simulink model "Quadcopter"  (R2019a)
settings: Solver=VariableStepAuto  StartTime=0.0  StopTime=2000  MaxStep=1e-1  RelTol=1e-3
StopFcn:
  | hold on;
  | plot3(out.out_y1.data, out.out_x1.data, out.out_z1.data, 'r');
  | plot3(out.out_y2.data, out.out_x2.data, out.out_z2.data, 'g');
  | plot3(out.out_y3.data, out.out_x3.data, out.out_z3.data, 'b');
  | plot3([0;out.out_y.data(1:1000:end)], [0;out.out_x.data(1:1000:end)], [0;out.out_z.data(1:1000:end)], '.k');
  | view(3);
  | hold off;
values from neighbouring files (symbols this model uses):
  B_phi = 1    [Control.m]
  B_psi = 1    [Control.m]
  B_theta = 1    [Control.m]
  B_z = 5    [Control.m]
  r_x12 = 8    [Control.m]
  r_x32 = 4    [Control.m]
  r_y12 = 8    [Control.m]
  r_y32 = 4    [Control.m]
undefined symbols (not defined in the file or in its folder): As, Bs, Cpsi, Cs, Cx, Cy, Cz, Ds, x01, x02, x03, y01, y02, y03, z01, z02, z03
libraries: simulink x1
(part 1 of 3)
settings Model: Creator=hvh  LastModifiedBy=hvh

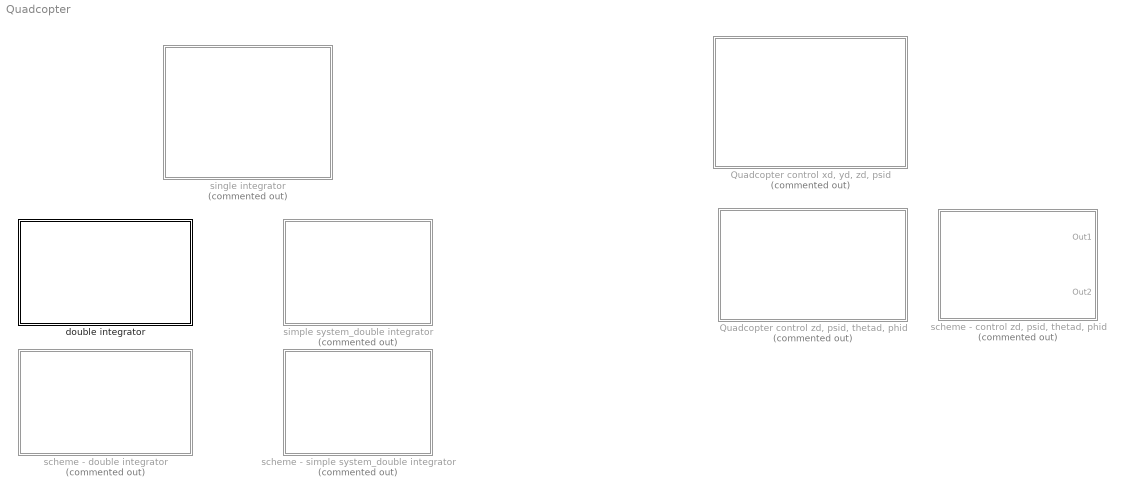
== system Quadcopter ==
  "Quadcopter control xd, yd, zd, psid" : Subsystem  Commented=on
  "Quadcopter control zd, psid, thetad, phid" : Subsystem  Commented=on
  double integrator : Subsystem
  "scheme - control zd, psid, thetad, phid" : Subsystem  Commented=on
  scheme - double integrator : Subsystem  Commented=on
  scheme - simple system_double integrator : Subsystem  Commented=on
  simple system_double integrator : Subsystem  Commented=on
  single integrator : Subsystem  Commented=on

== system Quadcopter/Quadcopter control xd, yd, zd, psid ==
  Controller : Subsystem
  Demux : Demux  Outputs=6
  Demux1 : Demux  Outputs=6
  Dynamic_System : Subsystem
  Mux : Mux  Inputs=6
  Mux1 : Mux  Inputs=6
  psi - psid : Scope  NumInputPorts=2
  psid : Step  Time=0  After=0.1  SampleTime=0
  x - xd : Scope  NumInputPorts=2
  xd : Step  Time=0  After=3  SampleTime=0
  y - yd : Scope  NumInputPorts=2
  yd : Step  Time=0  After=6  SampleTime=0
  z - zd : Scope  NumInputPorts=2
  zd : Step  Time=0  After=20  SampleTime=0
  wires:
  Dynamic_System/11(psi) -> Mux1/5
  Controller/4(tau_psi) -> Dynamic_System/4(tau_psi)
  Dynamic_System/3(y) -> Mux/3
  Dynamic_System/1(x) -> Mux/1
  Controller/2(tau_phi) -> Dynamic_System/2(tau_phi)
  Dynamic_System/5(z) -> Mux/5
  Controller/3(tau_theta) -> Dynamic_System/3(tau_theta)
  Controller/1(Ft) -> Dynamic_System/1(Ft)
  Dynamic_System/2(dx) -> Mux/2
  Dynamic_System/4(dy) -> Mux/4
  Dynamic_System/6(dz) -> Mux/6
  Dynamic_System/7(phi) -> Mux1/1
  Dynamic_System/8(dphi) -> Mux1/2
  Dynamic_System/9(theta) -> Mux1/3
  Dynamic_System/10(dtheta) -> Mux1/4
  Dynamic_System/12(dpsi) -> Mux1/6
  Demux/1 -> x - xd/1, Controller/1(x)
  Demux/2 -> Controller/2(dx)
  Demux/3 -> y - yd/1, Controller/3(y)
  Demux/4 -> Controller/4(dy)
  Demux/5 -> Controller/5(z), z - zd/1
  Demux/6 -> Controller/6(dz)
  Mux/1 -> Demux/1
  Demux1/2 -> Controller/8(dphi)
  Demux1/3 -> Controller/9(theta)
  Demux1/4 -> Controller/10(dtheta)
  Demux1/5 -> psi - psid/1, Controller/11(psi)
  Demux1/6 -> Controller/12(dpsi)
  Mux1/1 -> Demux1/1
  xd/1 -> x - xd/2, Controller/13(xd)
  yd/1 -> y - yd/2, Controller/14(yd)
  zd/1 -> z - zd/2, Controller/15(zd)
  psid/1 -> psi - psid/2, Controller/16(psid)
  Demux1/1 -> Controller/7(phi)

== system Quadcopter/Quadcopter control zd, psid, thetad, phid ==
  Controller : Subsystem
  Demux : Demux  Outputs=8
  Dynamic_System : Subsystem
  Mux : Mux  Inputs=8
  ddx : Scope
  ddy : Scope
  dphid : Step  Time=0  After=0  SampleTime=0
  dthetad : Step  Time=0  After=0  SampleTime=0
  dx : Scope
  dy : Scope
  phi : Scope  NumInputPorts=2
  phid : Step  Time=0  After=0.1  SampleTime=0
  psi : Scope  NumInputPorts=2
  psid : Step  Time=0  After=0.1  SampleTime=0
  theta : Scope  NumInputPorts=2
  thetad : Step  Time=0  After=0.15  SampleTime=0
  x : Scope
  y : Scope
  z : Scope  NumInputPorts=2
  zd : Step  Time=0  SampleTime=0
  wires:
  Dynamic_System/3(psi) -> Mux/3, psi/2
  Controller/4(tau_psi) -> Dynamic_System/4(tau_psi)
  Dynamic_System/12(y) -> y/1
  Dynamic_System/9(x) -> x/1
  Controller/2(tau_phi) -> Dynamic_System/2(tau_phi)
  Controller/3(tau_theta) -> Dynamic_System/3(tau_theta)
  Controller/1(Ft) -> Dynamic_System/1(Ft)
  Dynamic_System/10(dx) -> dx/1
  Dynamic_System/13(dy) -> dy/1
  Mux/1 -> Demux/1
  zd/1 -> z/1, Controller/9(zd)
  psid/1 -> psi/1, Controller/10(psid)
  phid/1 -> Controller/13(phid), phi/1
  dphid/1 -> Controller/14(dphid)
  thetad/1 -> Controller/11(thetad), theta/1
  dthetad/1 -> Controller/12(dthetad)
  Dynamic_System/11(ddx) -> ddx/1
  Dynamic_System/14(ddy) -> ddy/1
  Dynamic_System/1(z) -> z/2, Mux/1
  Dynamic_System/2(dz) -> Mux/2
  Dynamic_System/4(dpsi) -> Mux/4
  Dynamic_System/5(theta) -> theta/2, Mux/5
  Dynamic_System/6(dtheta) -> Mux/6
  Dynamic_System/8(dphi) -> Mux/8
  Dynamic_System/7(phi) -> Mux/7, phi/2
  Demux/1 -> Controller/1(z)
  Demux/2 -> Controller/2(dz)
  Demux/3 -> Controller/3(psi)
  Demux/4 -> Controller/4(dpsi)
  Demux/5 -> Controller/5(theta)
  Demux/6 -> Controller/6(dtheta)
  Demux/7 -> Controller/7(phi)
  Demux/8 -> Controller/8(dphi)

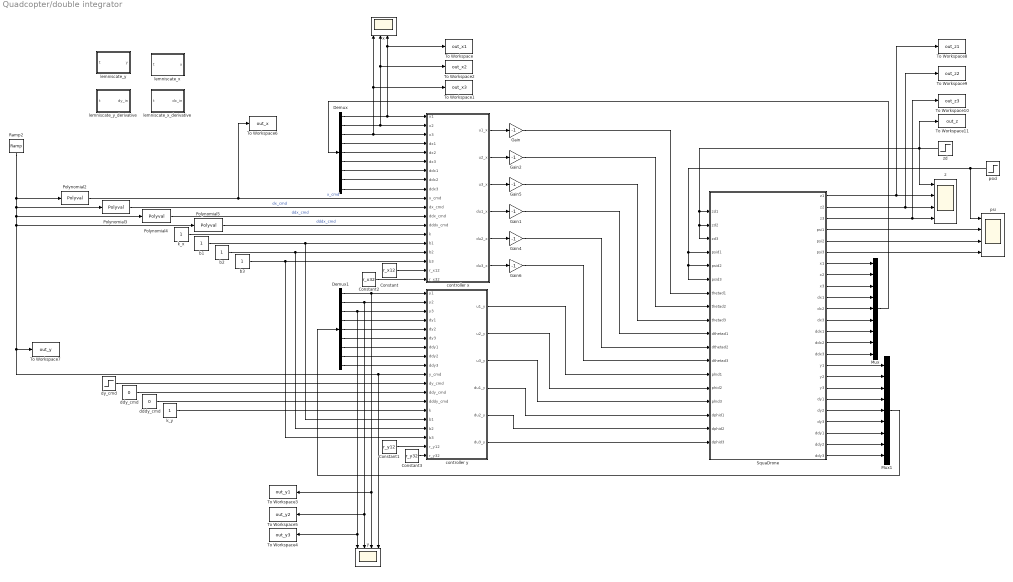
== system Quadcopter/double integrator ==
  Constant : Constant  Value=r_x12
  Constant1 : Constant  Value=r_y12
  Constant2 : Constant  Value=r_x32
  Constant3 : Constant  Value=r_y32
  Demux : Demux  Outputs=9
  Demux1 : Demux  Outputs=9
  Gain{,1..2,4..6} (6 alike) : Gain  Gain=-1
  Mux : Mux  Inputs=9
  Mux1 : Mux  Inputs=9
  Polynomial2 : Polyval  Coefs=[2*1e-5 -0.5*1e-2 0 0]
  Polynomial3 : Polyval  Coefs=[6*1e-5 -1e-2 0]
  Polynomial4 : Polyval  Coefs=[12*1e-5 -1e-2]
  Polynomial5 : Polyval  Coefs=[12*1e-5]
  Ramp2 : simulink/Sources/Ramp  slope=1/10  start=15  InitialOutput=0
  SquaDrone : Subsystem
  To Workspace : ToWorkspace  VariableName=out_x1  SaveFormat=Timeseries  SampleTime=-1
  To Workspace1 : ToWorkspace  VariableName=out_x3  SaveFormat=Timeseries  SampleTime=-1
  To Workspace10 : ToWorkspace  VariableName=out_z3  SaveFormat=Timeseries  SampleTime=-1
  To Workspace11 : ToWorkspace  VariableName=out_z  SaveFormat=Timeseries  SampleTime=-1
  To Workspace2 : ToWorkspace  VariableName=out_x2  SaveFormat=Timeseries  SampleTime=-1
  To Workspace3 : ToWorkspace  VariableName=out_y1  SaveFormat=Timeseries  SampleTime=-1
  To Workspace4 : ToWorkspace  VariableName=out_y3  SaveFormat=Timeseries  SampleTime=-1
  To Workspace5 : ToWorkspace  VariableName=out_y2  SaveFormat=Timeseries  SampleTime=-1
  To Workspace6 : ToWorkspace  VariableName=out_x  SaveFormat=Timeseries  SampleTime=-1
  To Workspace7 : ToWorkspace  VariableName=out_y  SaveFormat=Timeseries  SampleTime=-1
  To Workspace8 : ToWorkspace  VariableName=out_z1  SaveFormat=Timeseries  SampleTime=-1
  To Workspace9 : ToWorkspace  VariableName=out_z2  SaveFormat=Timeseries  SampleTime=-1
  b1 : Constant
  b2 : Constant
  b3 : Constant
  controller x : MATLAB Function  TreatAsAtomicUnit=on
  controller y : MATLAB Function  TreatAsAtomicUnit=on
  dddy_cmd : Constant  Value=0
  ddy_cmd : Constant  Value=0
  dy_cmd : Step  Time=15  SampleTime=0
  k_x : Constant
  k_y : Constant
  lemniscate_x : MATLAB Function  TreatAsAtomicUnit=on
  lemniscate_x_derivative : MATLAB Function  TreatAsAtomicUnit=on
  "lemniscate_y " : MATLAB Function  TreatAsAtomicUnit=on
  "lemniscate_y_derivative " : MATLAB Function  TreatAsAtomicUnit=on
  psi : Scope  NumInputPorts=4
  psid : Step  Time=0  After=0  SampleTime=0
  x : Scope  NumInputPorts=4
  y : Scope  NumInputPorts=4
  z : Scope  NumInputPorts=4
  zd : Step  Time=0  After=10  SampleTime=0
  wires:
  b2/1 -> controller x/16(b2), controller y/16(b2)
  b3/1 -> controller y/17(b3), controller x/17(b3)
  b1/1 -> controller x/15(b1), controller y/15(b1)
  k_x/1 -> controller x/14(k)
  controller x/1(u1_x) -> Gain/1
  controller x/4(du1_x) -> Gain1/1
  controller x/2(u2_x) -> Gain2/1
  controller x/5(du2_x) -> Gain4/1
  controller x/3(u3_x) -> Gain5/1
  controller x/6(du3_x) -> Gain6/1
  zd/1 -> To Workspace11/1, z/1, SquaDrone/3(zd3), SquaDrone/2(zd2), SquaDrone/1(zd1)
  psid/1 -> SquaDrone/6(psid3), SquaDrone/5(psid2), SquaDrone/4(psid1), psi/1
  Demux/5 -> controller x/5(dx2)
  Demux/6 -> controller x/6(dx3)
  Demux/8 -> controller x/8(ddx2)
  Demux/7 -> controller x/7(ddx1)
  Demux/9 -> controller x/9(ddx3)
  Demux1/4 -> controller y/4(dy1)
  Demux1/5 -> controller y/5(dy2)
  Demux1/6 -> controller y/6(dy3)
  Demux1/7 -> controller y/7(ddy1)
  Demux1/8 -> controller y/8(ddy2)
  Demux1/9 -> controller y/9(ddy3)
  Mux/1 -> Demux/1
  Demux/4 -> controller x/4(dx1)
  SquaDrone/10(dx1) -> Mux/4
  SquaDrone/11(dx2) -> Mux/5
  SquaDrone/12(dx3) -> Mux/6
  SquaDrone/13(ddx1) -> Mux/7
  SquaDrone/14(ddx2) -> Mux/8
  SquaDrone/15(ddx3) -> Mux/9
  SquaDrone/7(x1) -> Mux/1
  SquaDrone/8(x2) -> Mux/2
  SquaDrone/9(x3) -> Mux/3
  SquaDrone/23(ddy2) -> Mux1/8
  SquaDrone/24(ddy3) -> Mux1/9
  SquaDrone/22(ddy1) -> Mux1/7
  SquaDrone/21(dy3) -> Mux1/6
  SquaDrone/20(dy2) -> Mux1/5
  SquaDrone/19(dy1) -> Mux1/4
  SquaDrone/16(y1) -> Mux1/1
  SquaDrone/17(y2) -> Mux1/2
  SquaDrone/18(y3) -> Mux1/3
  Mux1/1 -> Demux1/1
  Demux/2 -> controller x/2(x2), x/2, To Workspace2/1
  Demux/3 -> controller x/3(x3), x/1, To Workspace1/1
  Demux/1 -> controller x/1(x1), x/3, To Workspace/1
  SquaDrone/6(psi3) -> psi/4
  SquaDrone/5(psi2) -> psi/3
  SquaDrone/4(psi1) -> psi/2
  SquaDrone/1(z1) -> To Workspace8/1, z/2
  SquaDrone/2(z2) -> To Workspace9/1, z/3
  SquaDrone/3(z3) -> To Workspace10/1, z/4
  Demux1/1 -> y/3, To Workspace3/1, controller y/1(y1)
  Demux1/2 -> y/2, To Workspace5/1, controller y/2(y2)
  Demux1/3 -> To Workspace4/1, y/1, controller y/3(y3)
  controller y/6(du3_y) -> SquaDrone/18(dphid3)
  controller y/5(du2_y) -> SquaDrone/17(dphid2)
  controller y/4(du1_y) -> SquaDrone/16(dphid1)
  controller y/3(u3_y) -> SquaDrone/15(phid3)
  controller y/2(u2_y) -> SquaDrone/14(phid2)
  controller y/1(u1_y) -> SquaDrone/13(phid1)
  Gain6/1 -> SquaDrone/12(dthetad3)
  Gain4/1 -> SquaDrone/11(dthetad2)
  Gain1/1 -> SquaDrone/10(dthetad1)
  Gain5/1 -> SquaDrone/9(thetad3)
  Gain2/1 -> SquaDrone/8(thetad2)
  Gain/1 -> SquaDrone/7(thetad1)
  Constant/1 -> controller x/18(r_x12)
  Constant1/1 -> controller y/18(r_y12)
  Constant2/1 -> controller x/19(r_x32)
  Constant3/1 -> controller y/19(r_y32)
  k_y/1 -> controller y/14(k)
  dy_cmd/1 -> controller y/11(dy_cmd)
  ddy_cmd/1 -> controller y/12(ddy_cmd)
  Polynomial2/1 -> To Workspace6/1, controller x/10(x_cmd)  "x_cmd"
  Polynomial3/1 -> controller x/11(dx_cmd)  "dx_cmd"
  Polynomial5/1 -> controller x/13(dddx_cmd)  "dddx_cmd"
  Polynomial4/1 -> controller x/12(ddx_cmd)  "ddx_cmd"
  Ramp2/1 -> To Workspace7/1, controller y/10(y_cmd), y/4, Polynomial5/1, Polynomial4/1, Polynomial3/1, Polynomial2/1
  dddy_cmd/1 -> controller y/13(dddy_cmd)

== system Quadcopter/scheme - control zd, psid, thetad, phid ==
  Controller : Subsystem
  Demux2 : Demux
  Desired input : Subsystem
  Drone : Subsystem
  Mux2 : Mux
  Out1 : Outport
  Out2 : Outport  Port=2
  wires:
  Demux2/1 -> Controller/1(In1)  "Z"
  Controller/1(Out1) -> Drone/1(In1)  "Ft"
  Controller/2(Out2) -> Drone/2(In2)  "tau_psi"
  Drone/4(Output3) -> Mux2/4  "PHI"
  Demux2/2 -> Controller/2(In2)  "PSI"
  Drone/1(Output) -> Mux2/1  "Z"
  Mux2/1 -> Demux2/1
  Demux2/3 -> Controller/3(In3)  "THETA"
  Controller/3(Out3) -> Drone/3(In3)  "tau_theta"
  Drone/3(Output2) -> Mux2/3  "THETA"
  Demux2/4 -> Controller/4(In4)  "PHI"
  Drone/2(Output1) -> Mux2/2  "PSI"
  Controller/4(Out4) -> Drone/4(In4)  "thau_phi"
  Drone/5(Output4) -> Out1/1  "X"
  Drone/6(Output5) -> Out2/1  "Y"
  Desired input/1(Out1) -> Controller/5(In5)  "Z_d"
  Desired input/2(Out2) -> Controller/6(In6)  "PSI_d"
  Desired input/3(Out3) -> Controller/7(In7)  "THETA_d"
  Desired input/4(Out4) -> Controller/8(In8)  "PHI_d"

== system Quadcopter/scheme - double integrator ==
  "Change input from (X,Y) to (THETA, PHI)" : MATLAB Function  TreatAsAtomicUnit=on
  Coefficients : Subsystem
  Desired Inputs of X_d and Y_d : Subsystem
  Desired Inputs of Z_d and PSI_d : Subsystem
  Distances : Subsystem
  SquaDrone : Subsystem
  controller x : MATLAB Function  TreatAsAtomicUnit=on
  controller y : MATLAB Function  TreatAsAtomicUnit=on
  wires:
  Desired Inputs of X_d and Y_d/1(X_d) -> controller x/2(X_dX_ddX_ddX_cmd)
  Desired Inputs of X_d and Y_d/2(Y_d) -> controller y/2(Y_dY_ddY_ddY_cmd)
  Coefficients/2(Coef_Y) -> controller y/3(k_b1_b2_b3)
  Coefficients/1(Coef_X) -> controller x/3(k_b1_b2_b3)
  Distances/1(Distance_X) -> controller x/4(r)
  Distances/2(Distance_Y) -> controller y/4(r)
  "Change input from (X,Y) to (THETA, PHI)"/1(THETA_d) -> SquaDrone/3(THETA_d)
  "Change input from (X,Y) to (THETA, PHI)"/2(dTHETA_d) -> SquaDrone/4(dTHETA_d)
  "Change input from (X,Y) to (THETA, PHI)"/3(PHI_d) -> SquaDrone/5(PHI_d)
  "Change input from (X,Y) to (THETA, PHI)"/4(dPHI_d) -> SquaDrone/6(dPHI_d)
  controller x/1(U_x) -> "Change input from (X,Y) to (THETA, PHI)"/1(U_x)
  controller x/2(dU_x) -> "Change input from (X,Y) to (THETA, PHI)"/2(dU_x)
  controller y/1(U_Y) -> "Change input from (X,Y) to (THETA, PHI)"/3(U_y)
  controller y/2(dU_Y) -> "Change input from (X,Y) to (THETA, PHI)"/4(dU_y)
  Desired Inputs of Z_d and PSI_d/1(Z_d) -> SquaDrone/1(Z_d)
  Desired Inputs of Z_d and PSI_d/2(PSI_d) -> SquaDrone/2(PSI_d)
  SquaDrone/1(X_dX_ddX) -> controller x/1(X_dX_ddX)
  SquaDrone/2(Y_dY_ddY) -> controller y/1(Y_dY_ddY)

== system Quadcopter/scheme - simple system_double integrator ==
  Coefficients : Subsystem
  Demux : Demux  Outputs=6
  Desired Inputs : Subsystem
  Distances : Subsystem
  Mux : Mux  Inputs=6
  "Path Tracking Controller " : MATLAB Function  TreatAsAtomicUnit=on
  System Dynamics : Subsystem
  wires:
  "Path Tracking Controller "/2(u2) -> System Dynamics/2(u2)  "u2"
  "Path Tracking Controller "/1(u1) -> System Dynamics/1(u1)  "u1"
  "Path Tracking Controller "/3(u3) -> System Dynamics/3(u3)  "u3"
  Demux/1 -> "Path Tracking Controller "/1(x1)
  Demux/2 -> "Path Tracking Controller "/2(dx1)
  Demux/3 -> "Path Tracking Controller "/3(x2)
  Demux/4 -> "Path Tracking Controller "/4(dx2)
  Demux/5 -> "Path Tracking Controller "/5(x3)
  Demux/6 -> "Path Tracking Controller "/6(dx3)
  System Dynamics/1(x1) -> Mux/1
  System Dynamics/2(dx1) -> Mux/2
  System Dynamics/3(x2) -> Mux/3
  System Dynamics/4(dx2) -> Mux/4
  System Dynamics/5(x3) -> Mux/5
  System Dynamics/6(dx3) -> Mux/6
  Mux/1 -> Demux/1
  Desired Inputs/1(x_cmd) -> "Path Tracking Controller "/7(x_cmd)
  Desired Inputs/2(dx_cmd) -> "Path Tracking Controller "/8(dx_cmd)
  Coefficients/1(k) -> "Path Tracking Controller "/9(k)
  Coefficients/2(b1) -> "Path Tracking Controller "/10(b1)
  Coefficients/3(b2) -> "Path Tracking Controller "/11(b2)
  Coefficients/4(b3) -> "Path Tracking Controller "/12(b3)
  Distances/1(r_12) -> "Path Tracking Controller "/13(r_12)
  Distances/2(r_32) -> "Path Tracking Controller "/14(r_32)

== system Quadcopter/simple system_double integrator ==
  Demux : Demux  Outputs=6
  Dynamics : Subsystem
  MATLAB Function : MATLAB Function  TreatAsAtomicUnit=on
  Mux : Mux  Inputs=6
  b{1..3,5} (4 alike) : Constant
  b4 : Constant  Value=2
  dx_cmd : Step  Time=0  After=0  SampleTime=0
  k : Constant
  x : Scope  NumInputPorts=4
  x_cmd : Step  Time=0  After=0  SampleTime=0
  wires:
  MATLAB Function/2(u2) -> Dynamics/2(u2)
  MATLAB Function/1(u1) -> Dynamics/1(u1)
  MATLAB Function/3(u3) -> Dynamics/3(u3)
  x_cmd/1 -> x/1, MATLAB Function/7(x_cmd)
  dx_cmd/1 -> MATLAB Function/8(dx_cmd)
  k/1 -> MATLAB Function/9(k)
  b1/1 -> MATLAB Function/10(b1)
  b2/1 -> MATLAB Function/11(b2)
  b3/1 -> MATLAB Function/12(b3)
  b4/1 -> MATLAB Function/13(r_12)
  b5/1 -> MATLAB Function/14(r_32)
  Dynamics/1(x1) -> x/2, Mux/1
  Dynamics/2(dx1) -> Mux/2
  Dynamics/3(x2) -> x/3, Mux/3
  Dynamics/4(dx2) -> Mux/4
  Dynamics/5(x3) -> x/4, Mux/5
  Dynamics/6(dx3) -> Mux/6
  Demux/1 -> MATLAB Function/1(x1)
  Demux/2 -> MATLAB Function/2(dx1)
  Demux/3 -> MATLAB Function/3(x2)
  Demux/4 -> MATLAB Function/4(dx2)
  Demux/5 -> MATLAB Function/5(x3)
  Demux/6 -> MATLAB Function/6(dx3)
  Mux/1 -> Demux/1

== system Quadcopter/single integrator ==
  Constant : Constant
  Constant1 : Constant
  Demux : Demux  Outputs=3
  Demux1 : Demux  Outputs=3
  Formation dynamics x : StateSpace  A=As  B=Bs  C=Cs  D=Ds  InitialCondition=0
  Formation dynamics y : StateSpace  A=As  B=Bs  C=Cs  D=Ds  InitialCondition=0
  SquaDrone : Subsystem
  psi : Scope  NumInputPorts=3
  psid : Step  Time=0  After=0.1  SampleTime=0
  u1_x = f() : MATLAB Function  TreatAsAtomicUnit=on
  u1_y = f() : MATLAB Function  TreatAsAtomicUnit=on
  x : Scope  NumInputPorts=3
  x_cmd : Step  Time=0  After=10  SampleTime=0
  y : Scope  NumInputPorts=3
  y_cmd : Step  Time=0  After=15  SampleTime=0
  z : Scope  NumInputPorts=3
  zd : Step  Time=0  After=50  SampleTime=0
  wires:
  SquaDrone/8(psi2) -> psi/2
  SquaDrone/11(z3) -> z/3
  Demux/2 -> SquaDrone/5(x2d)
  psid/1 -> SquaDrone/12(psi3d), SquaDrone/8(psi2d), SquaDrone/4(psi1d)
  Demux1/3 -> SquaDrone/10(y3d)
  Demux/3 -> SquaDrone/9(x3d)
  SquaDrone/5(x2) -> x/2, u1_x = f()/2(x2)
  zd/1 -> SquaDrone/3(z1d), SquaDrone/7(z2d), SquaDrone/11(z3d)
  Demux1/1 -> SquaDrone/2(y1d)
  Constant/1 -> u1_y = f()/5(k), u1_x = f()/5(k)
  Constant1/1 -> u1_y = f()/6(b), u1_x = f()/6(b)
  SquaDrone/1(x1) -> x/3, u1_x = f()/1(x1)
  Formation dynamics x/1 -> Demux/1
  SquaDrone/9(x3) -> u1_x = f()/3(x3), x/1
  SquaDrone/2(y1) -> y/3, u1_y = f()/1(y1)
  x_cmd/1 -> u1_x = f()/4(x_cmd)
  SquaDrone/6(y2) -> y/2, u1_y = f()/2(y2)
  SquaDrone/10(y3) -> y/1, u1_y = f()/3(y3)
  y_cmd/1 -> u1_y = f()/4(y_cmd)
  SquaDrone/3(z1) -> z/1
  SquaDrone/7(z2) -> z/2
  Demux1/2 -> SquaDrone/6(y2d)
  u1_x = f()/1(u1_x) -> Formation dynamics x/1
  Formation dynamics y/1 -> Demux1/1
  Demux/1 -> SquaDrone/1(x1d)
  u1_y = f()/1(u1_y) -> Formation dynamics y/1
  SquaDrone/4(psi1) -> psi/1
  SquaDrone/12(psi3) -> psi/3

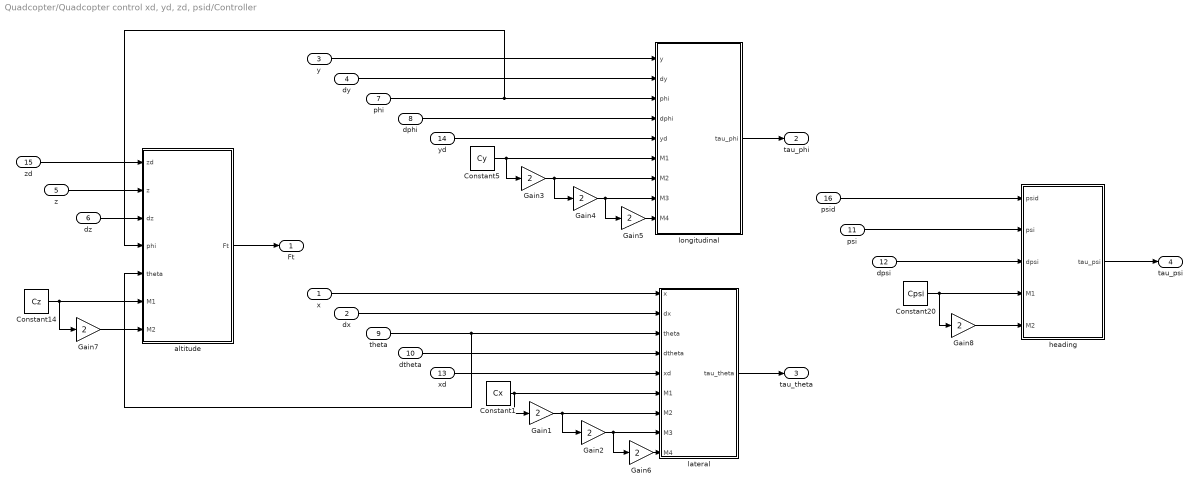
== system Quadcopter/Quadcopter control xd, yd, zd, psid/Controller ==
  x : Inport
  dx : Inport  Port=2
  y : Inport  Port=3
  dy : Inport  Port=4
  z : Inport  Port=5
  dz : Inport  Port=6
  phi : Inport  Port=7
  dphi : Inport  Port=8
  theta : Inport  Port=9
  dtheta : Inport  Port=10
  psi : Inport  Port=11
  dpsi : Inport  Port=12
  xd : Inport  Port=13
  yd : Inport  Port=14
  zd : Inport  Port=15
  psid : Inport  Port=16
  Constant1 : Constant  Value=Cx
  Constant14 : Constant  Value=Cz
  Constant20 : Constant  Value=Cpsi
  Constant5 : Constant  Value=Cy
  Gain{1..8} (8 alike) : Gain  Gain=2
  altitude : MATLAB Function  TreatAsAtomicUnit=on
  heading : MATLAB Function  TreatAsAtomicUnit=on
  lateral : MATLAB Function  TreatAsAtomicUnit=on
  longitudinal : MATLAB Function  TreatAsAtomicUnit=on
  Ft : Outport
  tau_phi : Outport  Port=2
  tau_theta : Outport  Port=3
  tau_psi : Outport  Port=4
  wires:
  altitude/1(Ft) -> Ft/1
  longitudinal/1(tau_phi) -> tau_phi/1
  lateral/1(tau_theta) -> tau_theta/1
  heading/1(tau_psi) -> tau_psi/1
  Gain7/1 -> altitude/7(M2)
  Constant14/1 -> Gain7/1, altitude/6(M1)
  Constant20/1 -> Gain8/1, heading/4(M1)
  Gain8/1 -> heading/5(M2)
  psid/1 -> heading/1(psid)
  psi/1 -> heading/2(psi)
  dpsi/1 -> heading/3(dpsi)
  dx/1 -> lateral/2(dx)
  x/1 -> lateral/1(x)
  theta/1 -> lateral/3(theta), altitude/5(theta)
  dtheta/1 -> lateral/4(dtheta)
  y/1 -> longitudinal/1(y)
  dy/1 -> longitudinal/2(dy)
  phi/1 -> altitude/4(phi), longitudinal/3(phi)
  dphi/1 -> longitudinal/4(dphi)
  xd/1 -> lateral/5(xd)
  yd/1 -> longitudinal/5(yd)
  zd/1 -> altitude/1(zd)
  z/1 -> altitude/2(z)
  dz/1 -> altitude/3(dz)
  Gain4/1 -> longitudinal/8(M3), Gain5/1
  Constant5/1 -> longitudinal/6(M1), Gain3/1
  Gain3/1 -> longitudinal/7(M2), Gain4/1
  Gain5/1 -> longitudinal/9(M4)
  Gain2/1 -> lateral/8(M3), Gain6/1
  Constant1/1 -> lateral/6(M1), Gain1/1
  Gain1/1 -> lateral/7(M2), Gain2/1
  Gain6/1 -> lateral/9(M4)

== system Quadcopter/Quadcopter control xd, yd, zd, psid/Dynamic_System ==
  Ft : Inport
  tau_phi : Inport  Port=2
  tau_theta : Inport  Port=3
  tau_psi : Inport  Port=4
  Demux : Demux  Outputs=3
  Integrator{,1..11} (12 alike) : Integrator
  MATLAB Function : MATLAB Function  TreatAsAtomicUnit=on
  MATLAB Function3 : MATLAB Function  TreatAsAtomicUnit=on
  MATLAB Function4 : MATLAB Function  TreatAsAtomicUnit=on
  Mux : Mux  Inputs=3
  x : Outport
  dx : Outport  Port=2
  y : Outport  Port=3
  dy : Outport  Port=4
  z : Outport  Port=5
  dz : Outport  Port=6
  phi : Outport  Port=7
  dphi : Outport  Port=8
  theta : Outport  Port=9
  dtheta : Outport  Port=10
  psi : Outport  Port=11
  dpsi : Outport  Port=12
  wires:
  MATLAB Function3/1(ddx) -> Integrator/1  "ddx"
  Ft/1 -> MATLAB Function3/1(Ft), MATLAB Function4/1(Ft), MATLAB Function/1(Ft)
  Integrator/1 -> dx/1, Integrator1/1  "dx"
  Integrator1/1 -> x/1  "x"
  MATLAB Function/1(ddy) -> Integrator2/1  "ddy"
  Integrator2/1 -> dy/1, Integrator3/1  "dy"
  Integrator3/1 -> y/1  "y"
  MATLAB Function4/1(ddz) -> Integrator4/1  "ddz"
  Integrator4/1 -> dz/1, Integrator5/1  "dz"
  Integrator5/1 -> z/1  "z"
  tau_phi/1 -> Integrator6/1  "ddphi"
  Integrator6/1 -> dphi/1, Integrator7/1  "dphi"
  Integrator7/1 -> Mux/1, phi/1  "phi"
  Integrator9/1 -> Mux/2, theta/1  "theta"
  Integrator8/1 -> dtheta/1, Integrator9/1  "dtheta"
  tau_theta/1 -> Integrator8/1  "ddtheta"
  Integrator11/1 -> Mux/3, psi/1  "psi"
  Integrator10/1 -> dpsi/1, Integrator11/1  "dpsi"
  tau_psi/1 -> Integrator10/1  "ddpsi"
  Mux/1 -> Demux/1  "(phi, theta, psi)"
  Demux/1 -> MATLAB Function3/2(phi), MATLAB Function4/2(phi), MATLAB Function/2(phi)
  Demux/2 -> MATLAB Function3/3(theta), MATLAB Function4/3(theta), MATLAB Function/3(theta)
  Demux/3 -> MATLAB Function/4(psi), MATLAB Function3/4(psi)

== system Quadcopter/Quadcopter control zd, psid, thetad, phid/Controller ==
  z : Inport
  dz : Inport  Port=2
  psi : Inport  Port=3
  dpsi : Inport  Port=4
  theta : Inport  Port=5
  dtheta : Inport  Port=6
  phi : Inport  Port=7
  dphi : Inport  Port=8
  zd : Inport  Port=9
  psid : Inport  Port=10
  thetad : Inport  Port=11
  dthetad : Inport  Port=12
  phid : Inport  Port=13
  dphid : Inport  Port=14
  Constant1 : Constant  Value=B_theta
  Constant14 : Constant  Value=B_z
  Constant20 : Constant  Value=B_psi
  Constant5 : Constant  Value=B_phi
  Gain{1,3,7..8} (4 alike) : Gain  Gain=2
  altitude : MATLAB Function  TreatAsAtomicUnit=on
  heading : MATLAB Function  TreatAsAtomicUnit=on
  lateral : MATLAB Function  TreatAsAtomicUnit=on
  longitudial : MATLAB Function  TreatAsAtomicUnit=on
  Ft : Outport
  tau_phi : Outport  Port=2
  tau_theta : Outport  Port=3
  tau_psi : Outport  Port=4
  wires:
  altitude/1(Ft) -> Ft/1
  longitudial/1(tau_phi) -> tau_phi/1
  lateral/1(tau_theta) -> tau_theta/1
  heading/1(tau_psi) -> tau_psi/1
  Gain7/1 -> altitude/7(M2)
  Constant14/1 -> Gain7/1, altitude/6(M1)
  Constant20/1 -> Gain8/1, heading/4(M1)
  Gain8/1 -> heading/5(M2)
  psid/1 -> heading/1(psid)
  psi/1 -> heading/2(psi)
  dpsi/1 -> heading/3(dpsi)
  theta/1 -> lateral/1(theta), altitude/4(theta)
  dtheta/1 -> lateral/2(dtheta)
  phi/1 -> longitudial/1(phi), altitude/3(phi)
  dphi/1 -> longitudial/2(dphi)
  zd/1 -> altitude/5(zd)
  z/1 -> altitude/1(z)
  dz/1 -> altitude/2(dz)
  Constant5/1 -> Gain3/1, longitudial/5(M1)
  Gain3/1 -> longitudial/6(M2)
  Constant1/1 -> Gain1/1, lateral/5(M1)
  Gain1/1 -> lateral/6(M2)
  thetad/1 -> lateral/3(thetad)
  dthetad/1 -> lateral/4(dthetad)
  phid/1 -> longitudial/3(phid)
  dphid/1 -> longitudial/4(dphid)

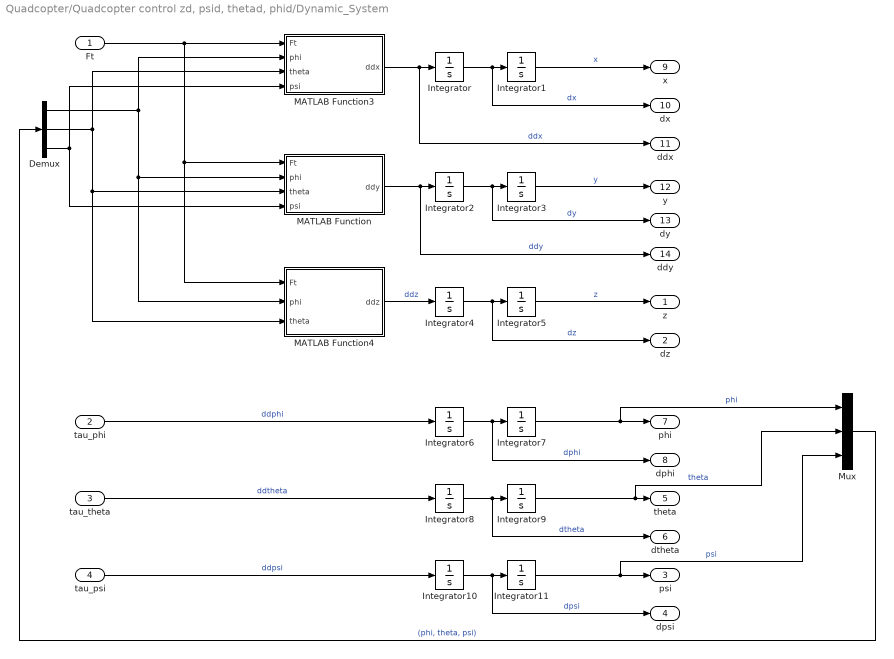
== system Quadcopter/Quadcopter control zd, psid, thetad, phid/Dynamic_System ==
  Ft : Inport
  tau_phi : Inport  Port=2
  tau_theta : Inport  Port=3
  tau_psi : Inport  Port=4
  Demux : Demux  Outputs=3
  Integrator{,1..11} (12 alike) : Integrator
  MATLAB Function : MATLAB Function  TreatAsAtomicUnit=on
  MATLAB Function3 : MATLAB Function  TreatAsAtomicUnit=on
  MATLAB Function4 : MATLAB Function  TreatAsAtomicUnit=on
  Mux : Mux  Inputs=3
  z : Outport
  dz : Outport  Port=2
  psi : Outport  Port=3
  dpsi : Outport  Port=4
  theta : Outport  Port=5
  dtheta : Outport  Port=6
  phi : Outport  Port=7
  dphi : Outport  Port=8
  x : Outport  Port=9
  dx : Outport  Port=10
  ddx : Outport  Port=11
  y : Outport  Port=12
  dy : Outport  Port=13
  ddy : Outport  Port=14
  wires:
  MATLAB Function3/1(ddx) -> ddx/1, Integrator/1  "ddx"
  Ft/1 -> MATLAB Function3/1(Ft), MATLAB Function4/1(Ft), MATLAB Function/1(Ft)
  Integrator/1 -> dx/1, Integrator1/1  "dx"
  Integrator1/1 -> x/1  "x"
  MATLAB Function/1(ddy) -> ddy/1, Integrator2/1  "ddy"
  Integrator2/1 -> dy/1, Integrator3/1  "dy"
  Integrator3/1 -> y/1  "y"
  MATLAB Function4/1(ddz) -> Integrator4/1  "ddz"
  Integrator4/1 -> dz/1, Integrator5/1  "dz"
  Integrator5/1 -> z/1  "z"
  tau_phi/1 -> Integrator6/1  "ddphi"
  Integrator6/1 -> dphi/1, Integrator7/1  "dphi"
  Integrator7/1 -> Mux/1, phi/1  "phi"
  Integrator9/1 -> Mux/2, theta/1  "theta"
  Integrator8/1 -> dtheta/1, Integrator9/1  "dtheta"
  tau_theta/1 -> Integrator8/1  "ddtheta"
  Integrator11/1 -> Mux/3, psi/1  "psi"
  Integrator10/1 -> dpsi/1, Integrator11/1  "dpsi"
  tau_psi/1 -> Integrator10/1  "ddpsi"
  Mux/1 -> Demux/1  "(phi, theta, psi)"
  Demux/1 -> MATLAB Function3/2(phi), MATLAB Function4/2(phi), MATLAB Function/2(phi)
  Demux/2 -> MATLAB Function3/3(theta), MATLAB Function4/3(theta), MATLAB Function/3(theta)
  Demux/3 -> MATLAB Function/4(psi), MATLAB Function3/4(psi)

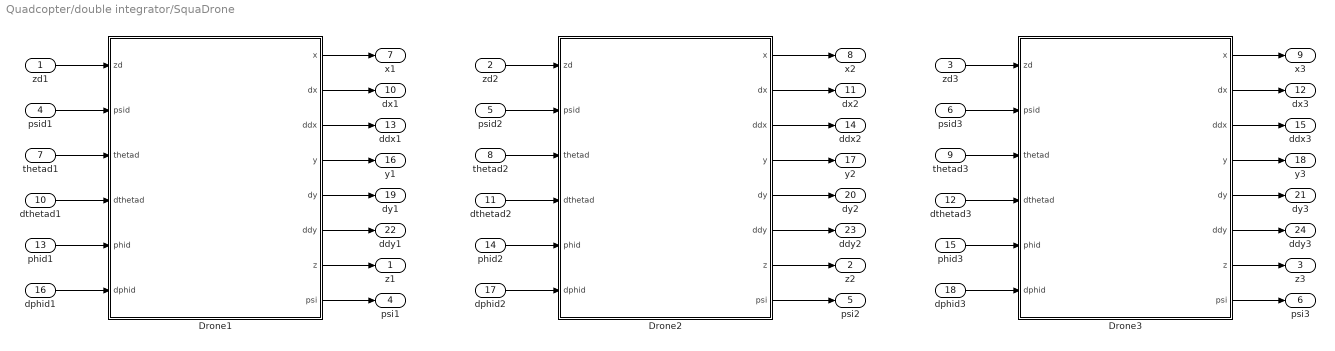
== system Quadcopter/double integrator/SquaDrone ==
  zd1 : Inport
  zd2 : Inport  Port=2
  zd3 : Inport  Port=3
  psid1 : Inport  Port=4
  psid2 : Inport  Port=5
  psid3 : Inport  Port=6
  thetad1 : Inport  Port=7
  thetad2 : Inport  Port=8
  thetad3 : Inport  Port=9
  dthetad1 : Inport  Port=10
  dthetad2 : Inport  Port=11
  dthetad3 : Inport  Port=12
  phid1 : Inport  Port=13
  phid2 : Inport  Port=14
  phid3 : Inport  Port=15
  dphid1 : Inport  Port=16
  dphid2 : Inport  Port=17
  dphid3 : Inport  Port=18
  Drone1 : Subsystem
  Drone2 : Subsystem
  Drone3 : Subsystem
  z1 : Outport
  z2 : Outport  Port=2
  z3 : Outport  Port=3
  psi1 : Outport  Port=4
  psi2 : Outport  Port=5
  psi3 : Outport  Port=6
  x1 : Outport  Port=7
  x2 : Outport  Port=8
  x3 : Outport  Port=9
  dx1 : Outport  Port=10
  dx2 : Outport  Port=11
  dx3 : Outport  Port=12
  ddx1 : Outport  Port=13
  ddx2 : Outport  Port=14
  ddx3 : Outport  Port=15
  y1 : Outport  Port=16
  y2 : Outport  Port=17
  y3 : Outport  Port=18
  dy1 : Outport  Port=19
  dy2 : Outport  Port=20
  dy3 : Outport  Port=21
  ddy1 : Outport  Port=22
  ddy2 : Outport  Port=23
  ddy3 : Outport  Port=24
  wires:
  Drone1/1(x) -> x1/1
  zd1/1 -> Drone1/1(zd)
  phid1/1 -> Drone1/5(phid)
  psid1/1 -> Drone1/2(psid)
  dphid1/1 -> Drone1/6(dphid)
  thetad1/1 -> Drone1/3(thetad)
  dthetad1/1 -> Drone1/4(dthetad)
  Drone1/2(dx) -> dx1/1
  Drone1/4(y) -> y1/1
  Drone1/5(dy) -> dy1/1
  Drone1/7(z) -> z1/1
  Drone1/8(psi) -> psi1/1
  Drone1/3(ddx) -> ddx1/1
  Drone1/6(ddy) -> ddy1/1
  zd2/1 -> Drone2/1(zd)
  psid2/1 -> Drone2/2(psid)
  dthetad2/1 -> Drone2/4(dthetad)
  phid2/1 -> Drone2/5(phid)
  thetad2/1 -> Drone2/3(thetad)
  dphid2/1 -> Drone2/6(dphid)
  zd3/1 -> Drone3/1(zd)
  psid3/1 -> Drone3/2(psid)
  dthetad3/1 -> Drone3/4(dthetad)
  phid3/1 -> Drone3/5(phid)
  thetad3/1 -> Drone3/3(thetad)
  dphid3/1 -> Drone3/6(dphid)
  Drone2/1(x) -> x2/1
  Drone2/2(dx) -> dx2/1
  Drone2/3(ddx) -> ddx2/1
  Drone2/4(y) -> y2/1
  Drone2/5(dy) -> dy2/1
  Drone2/6(ddy) -> ddy2/1
  Drone2/7(z) -> z2/1
  Drone2/8(psi) -> psi2/1
  Drone3/1(x) -> x3/1
  Drone3/2(dx) -> dx3/1
  Drone3/3(ddx) -> ddx3/1
  Drone3/4(y) -> y3/1
  Drone3/5(dy) -> dy3/1
  Drone3/6(ddy) -> ddy3/1
  Drone3/7(z) -> z3/1
  Drone3/8(psi) -> psi3/1

== system Quadcopter/scheme - control zd, psid, thetad, phid/Controller ==
  In1 : Inport
  In2 : Inport  Port=2
  In3 : Inport  Port=3
  In4 : Inport  Port=4
  In5 : Inport  Port=5
  In6 : Inport  Port=6
  In7 : Inport  Port=7
  In8 : Inport  Port=8
  Out1 : Outport
  Out2 : Outport  Port=2
  Out3 : Outport  Port=3
  Out4 : Outport  Port=4

== system Quadcopter/scheme - control zd, psid, thetad, phid/Desired input ==
  Out1 : Outport
  Out2 : Outport  Port=2
  Out3 : Outport  Port=3
  Out4 : Outport  Port=4

== system Quadcopter/scheme - control zd, psid, thetad, phid/Drone ==
  In1 : Inport
  In2 : Inport  Port=2
  In3 : Inport  Port=3
  In4 : Inport  Port=4
  Output : Outport
  Output1 : Outport  Port=2
  Output2 : Outport  Port=3
  Output3 : Outport  Port=4
  Output4 : Outport  Port=5
  Output5 : Outport  Port=6

== system Quadcopter/scheme - double integrator/Coefficients ==
  Coef_X : Outport
  Coef_Y : Outport  Port=2

== system Quadcopter/scheme - double integrator/Desired Inputs of X_d and Y_d ==
  X_d : Outport
  Y_d : Outport  Port=2

== system Quadcopter/scheme - double integrator/Desired Inputs of Z_d and PSI_d ==
  Z_d : Outport
  PSI_d : Outport  Port=2

== system Quadcopter/scheme - double integrator/Distances ==
  Distance_X : Outport
  Distance_Y : Outport  Port=2

== system Quadcopter/scheme - double integrator/SquaDrone ==
  Z_d : Inport
  PSI_d : Inport  Port=2
  THETA_d : Inport  Port=3
  dTHETA_d : Inport  Port=4
  PHI_d : Inport  Port=5
  dPHI_d : Inport  Port=6
  Drone1 : Subsystem
  Drone2 : Subsystem
  Drone3 : Subsystem
  X_dX_ddX : Outport
  Y_dY_ddY : Outport  Port=2

== system Quadcopter/scheme - simple system_double integrator/Coefficients ==
  k : Outport
  b1 : Outport  Port=2
  b2 : Outport  Port=3
  b3 : Outport  Port=4

== system Quadcopter/scheme - simple system_double integrator/Desired Inputs ==
  x_cmd : Outport
  dx_cmd : Outport  Port=2

== system Quadcopter/scheme - simple system_double integrator/Distances ==
  r_12 : Outport
  r_32 : Outport  Port=2

== system Quadcopter/scheme - simple system_double integrator/System Dynamics ==
  u1 : Inport
  u2 : Inport  Port=2
  u3 : Inport  Port=3
  x1 : Outport
  dx1 : Outport  Port=2
  x2 : Outport  Port=3
  dx2 : Outport  Port=4
  x3 : Outport  Port=5
  dx3 : Outport  Port=6

== system Quadcopter/simple system_double integrator/Dynamics ==
  u1 : Inport
  u2 : Inport  Port=2
  u3 : Inport  Port=3
  Integrator{,1..5} (6 alike) : Integrator
  x1 : Outport
  dx1 : Outport  Port=2
  x2 : Outport  Port=3
  dx2 : Outport  Port=4
  x3 : Outport  Port=5
  dx3 : Outport  Port=6
  wires:
  u1/1 -> Integrator/1
  Integrator1/1 -> x1/1
  Integrator/1 -> dx1/1, Integrator1/1
  Integrator3/1 -> x2/1
  Integrator2/1 -> dx2/1, Integrator3/1
  Integrator5/1 -> x3/1
  Integrator4/1 -> dx3/1, Integrator5/1
  u3/1 -> Integrator4/1
  u2/1 -> Integrator2/1

== system Quadcopter/single integrator/SquaDrone ==
  x1d : Inport
  y1d : Inport  Port=2
  z1d : Inport  Port=3
  psi1d : Inport  Port=4
  x2d : Inport  Port=5
  y2d : Inport  Port=6
  z2d : Inport  Port=7
  psi2d : Inport  Port=8
  x3d : Inport  Port=9
  y3d : Inport  Port=10
  z3d : Inport  Port=11
  psi3d : Inport  Port=12
  Quadcopter1 : Subsystem
  Quadcopter2 : Subsystem
  Quadcopter3 : Subsystem
  x1 : Outport
  y1 : Outport  Port=2
  z1 : Outport  Port=3
  psi1 : Outport  Port=4
  x2 : Outport  Port=5
  y2 : Outport  Port=6
  z2 : Outport  Port=7
  psi2 : Outport  Port=8
  x3 : Outport  Port=9
  y3 : Outport  Port=10
  z3 : Outport  Port=11
  psi3 : Outport  Port=12
  wires:
  Quadcopter2/3(z) -> z2/1
  Quadcopter3/2(y) -> y3/1
  Quadcopter1/1(x) -> x1/1
  Quadcopter3/4(psi) -> psi3/1
  x1d/1 -> Quadcopter1/1(xd)
  Quadcopter1/2(y) -> y1/1
  Quadcopter2/4(psi) -> psi2/1
  Quadcopter2/2(y) -> y2/1
  y3d/1 -> Quadcopter3/2(yd)
  y2d/1 -> Quadcopter2/2(yd)
  Quadcopter2/1(x) -> x2/1
  Quadcopter3/1(x) -> x3/1
  psi3d/1 -> Quadcopter3/4(psid)
  y1d/1 -> Quadcopter1/2(yd)
  z2d/1 -> Quadcopter2/3(zd)
  z3d/1 -> Quadcopter3/3(zd)
  Quadcopter3/3(z) -> z3/1
  x3d/1 -> Quadcopter3/1(xd)
  Quadcopter1/3(z) -> z1/1
  Quadcopter1/4(psi) -> psi1/1
  x2d/1 -> Quadcopter2/1(xd)
  psi2d/1 -> Quadcopter2/4(psid)
  z1d/1 -> Quadcopter1/3(zd)
  psi1d/1 -> Quadcopter1/4(psid)

== system Quadcopter/double integrator/SquaDrone/Drone1 ==
  zd : Inport
  psid : Inport  Port=2
  thetad : Inport  Port=3
  dthetad : Inport  Port=4
  phid : Inport  Port=5
  dphid : Inport  Port=6
  Controller : Subsystem
  Demux : Demux  Outputs=8
  Dynamic_System : Subsystem
  Mux : Mux  Inputs=8
  Scope : Scope  NumInputPorts=2
  x : Outport
  dx : Outport  Port=2
  ddx : Outport  Port=3
  y : Outport  Port=4
  dy : Outport  Port=5
  ddy : Outport  Port=6
  z : Outport  Port=7
  psi : Outport  Port=8
  wires:
  Dynamic_System/3(psi) -> psi/1, Mux/3
  Controller/4(tau_psi) -> Dynamic_System/4(tau_psi)
  Controller/2(tau_phi) -> Dynamic_System/2(tau_phi)
  Controller/3(tau_theta) -> Dynamic_System/3(tau_theta)
  Controller/1(Ft) -> Dynamic_System/1(Ft)
  Mux/1 -> Demux/1
  Dynamic_System/14(ddy) -> ddy/1
  Dynamic_System/1(z) -> z/1, Mux/1
  Dynamic_System/2(dz) -> Mux/2
  Dynamic_System/4(dpsi) -> Mux/4
  Dynamic_System/5(theta) -> Scope/1, Mux/5
  Dynamic_System/6(dtheta) -> Mux/6
  Dynamic_System/8(dphi) -> Mux/8
  Dynamic_System/7(phi) -> Scope/2, Mux/7
  Demux/1 -> Controller/1(z)
  Demux/2 -> Controller/2(dz)
  Demux/3 -> Controller/3(psi)
  Demux/4 -> Controller/4(dpsi)
  Demux/5 -> Controller/5(theta)
  Demux/6 -> Controller/6(dtheta)
  Demux/7 -> Controller/7(phi)
  Demux/8 -> Controller/8(dphi)
  thetad/1 -> Controller/11(thetad)
  dthetad/1 -> Controller/12(dthetad)
  dphid/1 -> Controller/14(dphid)
  zd/1 -> Controller/9(zd)
  psid/1 -> Controller/10(psid)
  phid/1 -> Controller/13(phid)
  Dynamic_System/9(x) -> x/1
  Dynamic_System/10(dx) -> dx/1
  Dynamic_System/11(ddx) -> ddx/1
  Dynamic_System/12(y) -> y/1
  Dynamic_System/13(dy) -> dy/1

== system Quadcopter/double integrator/SquaDrone/Drone2 ==
  zd : Inport
  psid : Inport  Port=2
  thetad : Inport  Port=3
  dthetad : Inport  Port=4
  phid : Inport  Port=5
  dphid : Inport  Port=6
  Controller : Subsystem
  Demux : Demux  Outputs=8
  Dynamic_System : Subsystem
  Mux : Mux  Inputs=8
  x : Outport
  dx : Outport  Port=2
  ddx : Outport  Port=3
  y : Outport  Port=4
  dy : Outport  Port=5
  ddy : Outport  Port=6
  z : Outport  Port=7
  psi : Outport  Port=8
  wires:
  Dynamic_System/3(psi) -> psi/1, Mux/3
  Controller/4(tau_psi) -> Dynamic_System/4(tau_psi)
  Controller/2(tau_phi) -> Dynamic_System/2(tau_phi)
  Controller/3(tau_theta) -> Dynamic_System/3(tau_theta)
  Controller/1(Ft) -> Dynamic_System/1(Ft)
  Mux/1 -> Demux/1
  Dynamic_System/14(ddy) -> ddy/1
  Dynamic_System/1(z) -> z/1, Mux/1
  Dynamic_System/2(dz) -> Mux/2
  Dynamic_System/4(dpsi) -> Mux/4
  Dynamic_System/5(theta) -> Mux/5
  Dynamic_System/6(dtheta) -> Mux/6
  Dynamic_System/8(dphi) -> Mux/8
  Dynamic_System/7(phi) -> Mux/7
  Demux/1 -> Controller/1(z)
  Demux/2 -> Controller/2(dz)
  Demux/3 -> Controller/3(psi)
  Demux/4 -> Controller/4(dpsi)
  Demux/5 -> Controller/5(theta)
  Demux/6 -> Controller/6(dtheta)
  Demux/7 -> Controller/7(phi)
  Demux/8 -> Controller/8(dphi)
  thetad/1 -> Controller/11(thetad)
  dthetad/1 -> Controller/12(dthetad)
  dphid/1 -> Controller/14(dphid)
  zd/1 -> Controller/9(zd)
  psid/1 -> Controller/10(psid)
  phid/1 -> Controller/13(phid)
  Dynamic_System/9(x) -> x/1
  Dynamic_System/10(dx) -> dx/1
  Dynamic_System/11(ddx) -> ddx/1
  Dynamic_System/12(y) -> y/1
  Dynamic_System/13(dy) -> dy/1

== system Quadcopter/double integrator/SquaDrone/Drone3 ==
  zd : Inport
  psid : Inport  Port=2
  thetad : Inport  Port=3
  dthetad : Inport  Port=4
  phid : Inport  Port=5
  dphid : Inport  Port=6
  Controller : Subsystem
  Demux : Demux  Outputs=8
  Dynamic_System : Subsystem
  Mux : Mux  Inputs=8
  x : Outport
  dx : Outport  Port=2
  ddx : Outport  Port=3
  y : Outport  Port=4
  dy : Outport  Port=5
  ddy : Outport  Port=6
  z : Outport  Port=7
  psi : Outport  Port=8
  wires:
  Dynamic_System/3(psi) -> psi/1, Mux/3
  Controller/4(tau_psi) -> Dynamic_System/4(tau_psi)
  Controller/2(tau_phi) -> Dynamic_System/2(tau_phi)
  Controller/3(tau_theta) -> Dynamic_System/3(tau_theta)
  Controller/1(Ft) -> Dynamic_System/1(Ft)
  Mux/1 -> Demux/1
  Dynamic_System/14(ddy) -> ddy/1
  Dynamic_System/1(z) -> z/1, Mux/1
  Dynamic_System/2(dz) -> Mux/2
  Dynamic_System/4(dpsi) -> Mux/4
  Dynamic_System/5(theta) -> Mux/5
  Dynamic_System/6(dtheta) -> Mux/6
  Dynamic_System/8(dphi) -> Mux/8
  Dynamic_System/7(phi) -> Mux/7
  Demux/1 -> Controller/1(z)
  Demux/2 -> Controller/2(dz)
  Demux/3 -> Controller/3(psi)
  Demux/4 -> Controller/4(dpsi)
  Demux/5 -> Controller/5(theta)
  Demux/6 -> Controller/6(dtheta)
  Demux/7 -> Controller/7(phi)
  Demux/8 -> Controller/8(dphi)
  thetad/1 -> Controller/11(thetad)
  dthetad/1 -> Controller/12(dthetad)
  dphid/1 -> Controller/14(dphid)
  zd/1 -> Controller/9(zd)
  psid/1 -> Controller/10(psid)
  phid/1 -> Controller/13(phid)
  Dynamic_System/9(x) -> x/1
  Dynamic_System/10(dx) -> dx/1
  Dynamic_System/11(ddx) -> ddx/1
  Dynamic_System/12(y) -> y/1
  Dynamic_System/13(dy) -> dy/1

== system Quadcopter/scheme - double integrator/SquaDrone/Drone1 ==
  zd : Inport
  psid : Inport  Port=2
  thetad : Inport  Port=3
  dthetad : Inport  Port=4
  phid : Inport  Port=5
  dphid : Inport  Port=6
  Controller : Subsystem
  Demux : Demux  Outputs=8
  Dynamic_System : Subsystem
  Mux : Mux  Inputs=8
  Scope : Scope  NumInputPorts=2
  x : Outport
  dx : Outport  Port=2
  ddx : Outport  Port=3
  y : Outport  Port=4
  dy : Outport  Port=5
  ddy : Outport  Port=6
  z : Outport  Port=7
  psi : Outport  Port=8
  wires:
  Dynamic_System/3(psi) -> psi/1, Mux/3
  Controller/4(tau_psi) -> Dynamic_System/4(tau_psi)
  Controller/2(tau_phi) -> Dynamic_System/2(tau_phi)
  Controller/3(tau_theta) -> Dynamic_System/3(tau_theta)
  Controller/1(Ft) -> Dynamic_System/1(Ft)
  Mux/1 -> Demux/1
  Dynamic_System/14(ddy) -> ddy/1
  Dynamic_System/1(z) -> z/1, Mux/1
  Dynamic_System/2(dz) -> Mux/2
  Dynamic_System/4(dpsi) -> Mux/4
  Dynamic_System/5(theta) -> Scope/1, Mux/5
  Dynamic_System/6(dtheta) -> Mux/6
  Dynamic_System/8(dphi) -> Mux/8
  Dynamic_System/7(phi) -> Scope/2, Mux/7
  Demux/1 -> Controller/1(z)
  Demux/2 -> Controller/2(dz)
  Demux/3 -> Controller/3(psi)
  Demux/4 -> Controller/4(dpsi)
  Demux/5 -> Controller/5(theta)
  Demux/6 -> Controller/6(dtheta)
  Demux/7 -> Controller/7(phi)
  Demux/8 -> Controller/8(dphi)
  thetad/1 -> Controller/11(thetad)
  dthetad/1 -> Controller/12(dthetad)
  dphid/1 -> Controller/14(dphid)
  zd/1 -> Controller/9(zd)
  psid/1 -> Controller/10(psid)
  phid/1 -> Controller/13(phid)
  Dynamic_System/9(x) -> x/1
  Dynamic_System/10(dx) -> dx/1
  Dynamic_System/11(ddx) -> ddx/1
  Dynamic_System/12(y) -> y/1
  Dynamic_System/13(dy) -> dy/1

== system Quadcopter/scheme - double integrator/SquaDrone/Drone2 ==
  zd : Inport
  psid : Inport  Port=2
  thetad : Inport  Port=3
  dthetad : Inport  Port=4
  phid : Inport  Port=5
  dphid : Inport  Port=6
  Controller : Subsystem
  Demux : Demux  Outputs=8
  Dynamic_System : Subsystem
  Mux : Mux  Inputs=8
  Scope : Scope  NumInputPorts=2
  x : Outport
  dx : Outport  Port=2
  ddx : Outport  Port=3
  y : Outport  Port=4
  dy : Outport  Port=5
  ddy : Outport  Port=6
  z : Outport  Port=7
  psi : Outport  Port=8
  wires:
  Dynamic_System/3(psi) -> psi/1, Mux/3
  Controller/4(tau_psi) -> Dynamic_System/4(tau_psi)
  Controller/2(tau_phi) -> Dynamic_System/2(tau_phi)
  Controller/3(tau_theta) -> Dynamic_System/3(tau_theta)
  Controller/1(Ft) -> Dynamic_System/1(Ft)
  Mux/1 -> Demux/1
  Dynamic_System/14(ddy) -> ddy/1
  Dynamic_System/1(z) -> z/1, Mux/1
  Dynamic_System/2(dz) -> Mux/2
  Dynamic_System/4(dpsi) -> Mux/4
  Dynamic_System/5(theta) -> Scope/1, Mux/5
  Dynamic_System/6(dtheta) -> Mux/6
  Dynamic_System/8(dphi) -> Mux/8
  Dynamic_System/7(phi) -> Scope/2, Mux/7
  Demux/1 -> Controller/1(z)
  Demux/2 -> Controller/2(dz)
  Demux/3 -> Controller/3(psi)
  Demux/4 -> Controller/4(dpsi)
  Demux/5 -> Controller/5(theta)
  Demux/6 -> Controller/6(dtheta)
  Demux/7 -> Controller/7(phi)
  Demux/8 -> Controller/8(dphi)
  thetad/1 -> Controller/11(thetad)
  dthetad/1 -> Controller/12(dthetad)
  dphid/1 -> Controller/14(dphid)
  zd/1 -> Controller/9(zd)
  psid/1 -> Controller/10(psid)
  phid/1 -> Controller/13(phid)
  Dynamic_System/9(x) -> x/1
  Dynamic_System/10(dx) -> dx/1
  Dynamic_System/11(ddx) -> ddx/1
  Dynamic_System/12(y) -> y/1
  Dynamic_System/13(dy) -> dy/1

== system Quadcopter/scheme - double integrator/SquaDrone/Drone3 ==
  zd : Inport
  psid : Inport  Port=2
  thetad : Inport  Port=3
  dthetad : Inport  Port=4
  phid : Inport  Port=5
  dphid : Inport  Port=6
  Controller : Subsystem
  Demux : Demux  Outputs=8
  Dynamic_System : Subsystem
  Mux : Mux  Inputs=8
  Scope : Scope  NumInputPorts=2
  x : Outport
  dx : Outport  Port=2
  ddx : Outport  Port=3
  y : Outport  Port=4
  dy : Outport  Port=5
  ddy : Outport  Port=6
  z : Outport  Port=7
  psi : Outport  Port=8
  wires:
  Dynamic_System/3(psi) -> psi/1, Mux/3
  Controller/4(tau_psi) -> Dynamic_System/4(tau_psi)
  Controller/2(tau_phi) -> Dynamic_System/2(tau_phi)
  Controller/3(tau_theta) -> Dynamic_System/3(tau_theta)
  Controller/1(Ft) -> Dynamic_System/1(Ft)
  Mux/1 -> Demux/1
  Dynamic_System/14(ddy) -> ddy/1
  Dynamic_System/1(z) -> z/1, Mux/1
  Dynamic_System/2(dz) -> Mux/2
  Dynamic_System/4(dpsi) -> Mux/4
  Dynamic_System/5(theta) -> Scope/1, Mux/5
  Dynamic_System/6(dtheta) -> Mux/6
  Dynamic_System/8(dphi) -> Mux/8
  Dynamic_System/7(phi) -> Scope/2, Mux/7
  Demux/1 -> Controller/1(z)
  Demux/2 -> Controller/2(dz)
  Demux/3 -> Controller/3(psi)
  Demux/4 -> Controller/4(dpsi)
  Demux/5 -> Controller/5(theta)
  Demux/6 -> Controller/6(dtheta)
  Demux/7 -> Controller/7(phi)
  Demux/8 -> Controller/8(dphi)
  thetad/1 -> Controller/11(thetad)
  dthetad/1 -> Controller/12(dthetad)
  dphid/1 -> Controller/14(dphid)
  zd/1 -> Controller/9(zd)
  psid/1 -> Controller/10(psid)
  phid/1 -> Controller/13(phid)
  Dynamic_System/9(x) -> x/1
  Dynamic_System/10(dx) -> dx/1
  Dynamic_System/11(ddx) -> ddx/1
  Dynamic_System/12(y) -> y/1
  Dynamic_System/13(dy) -> dy/1

== system Quadcopter/single integrator/SquaDrone/Quadcopter1 ==
  xd : Inport
  yd : Inport  Port=2
  zd : Inport  Port=3
  psid : Inport  Port=4
  Controller : Subsystem
  Demux : Demux  Outputs=6
  Demux1 : Demux  Outputs=6
  Dynamic_System : Subsystem
  Mux : Mux  Inputs=6
  Mux1 : Mux  Inputs=6
  psi - psid : Scope  NumInputPorts=2
  x - xd : Scope  NumInputPorts=2
  y - yd : Scope  NumInputPorts=2
  z - zd : Scope  NumInputPorts=2
  x : Outport
  y : Outport  Port=2
  z : Outport  Port=3
  psi : Outport  Port=4
  wires:
  Dynamic_System/11(psi) -> psi/1, Mux1/5
  Controller/4(tau_psi) -> Dynamic_System/4(tau_psi)
  Dynamic_System/3(y) -> y/1, Mux/3
  Dynamic_System/1(x) -> x/1, Mux/1
  Controller/2(tau_phi) -> Dynamic_System/2(tau_phi)
  Dynamic_System/5(z) -> z/1, Mux/5
  Controller/3(tau_theta) -> Dynamic_System/3(tau_theta)
  Controller/1(Ft) -> Dynamic_System/1(Ft)
  Dynamic_System/2(dx) -> Mux/2
  Dynamic_System/4(dy) -> Mux/4
  Dynamic_System/6(dz) -> Mux/6
  Dynamic_System/7(phi) -> Mux1/1
  Dynamic_System/8(dphi) -> Mux1/2
  Dynamic_System/9(theta) -> Mux1/3
  Dynamic_System/10(dtheta) -> Mux1/4
  Dynamic_System/12(dpsi) -> Mux1/6
  Demux/1 -> x - xd/1, Controller/1(x)
  Demux/2 -> Controller/2(dx)
  Demux/3 -> y - yd/1, Controller/3(y)
  Demux/4 -> Controller/4(dy)
  Demux/5 -> Controller/5(z), z - zd/1
  Demux/6 -> Controller/6(dz)
  Mux/1 -> Demux/1
  Demux1/2 -> Controller/8(dphi)
  Demux1/3 -> Controller/9(theta)
  Demux1/4 -> Controller/10(dtheta)
  Demux1/5 -> psi - psid/1, Controller/11(psi)
  Demux1/6 -> Controller/12(dpsi)
  Mux1/1 -> Demux1/1
  xd/1 -> x - xd/2, Controller/13(xd)
  yd/1 -> y - yd/2, Controller/14(yd)
  zd/1 -> z - zd/2, Controller/15(zd)
  psid/1 -> psi - psid/2, Controller/16(psid)
  Demux1/1 -> Controller/7(phi)

== system Quadcopter/single integrator/SquaDrone/Quadcopter2 ==
  xd : Inport
  yd : Inport  Port=2
  zd : Inport  Port=3
  psid : Inport  Port=4
  Controller : Subsystem
  Demux : Demux  Outputs=6
  Demux1 : Demux  Outputs=6
  Dynamic_System : Subsystem
  Mux : Mux  Inputs=6
  Mux1 : Mux  Inputs=6
  psi - psid : Scope  NumInputPorts=2
  x - xd : Scope  NumInputPorts=2
  y - yd : Scope  NumInputPorts=2
  z - zd : Scope  NumInputPorts=2
  x : Outport
  y : Outport  Port=2
  z : Outport  Port=3
  psi : Outport  Port=4
  wires:
  Dynamic_System/11(psi) -> psi/1, Mux1/5
  Controller/4(tau_psi) -> Dynamic_System/4(tau_psi)
  Dynamic_System/3(y) -> y/1, Mux/3
  Dynamic_System/1(x) -> x/1, Mux/1
  Controller/2(tau_phi) -> Dynamic_System/2(tau_phi)
  Dynamic_System/5(z) -> z/1, Mux/5
  Controller/3(tau_theta) -> Dynamic_System/3(tau_theta)
  Controller/1(Ft) -> Dynamic_System/1(Ft)
  Dynamic_System/2(dx) -> Mux/2
  Dynamic_System/4(dy) -> Mux/4
  Dynamic_System/6(dz) -> Mux/6
  Dynamic_System/7(phi) -> Mux1/1
  Dynamic_System/8(dphi) -> Mux1/2
  Dynamic_System/9(theta) -> Mux1/3
  Dynamic_System/10(dtheta) -> Mux1/4
  Dynamic_System/12(dpsi) -> Mux1/6
  Demux/1 -> x - xd/1, Controller/1(x)
  Demux/2 -> Controller/2(dx)
  Demux/3 -> y - yd/1, Controller/3(y)
  Demux/4 -> Controller/4(dy)
  Demux/5 -> Controller/5(z), z - zd/1
  Demux/6 -> Controller/6(dz)
  Mux/1 -> Demux/1
  Demux1/2 -> Controller/8(dphi)
  Demux1/3 -> Controller/9(theta)
  Demux1/4 -> Controller/10(dtheta)
  Demux1/5 -> psi - psid/1, Controller/11(psi)
  Demux1/6 -> Controller/12(dpsi)
  Mux1/1 -> Demux1/1
  xd/1 -> x - xd/2, Controller/13(xd)
  yd/1 -> y - yd/2, Controller/14(yd)
  zd/1 -> z - zd/2, Controller/15(zd)
  psid/1 -> psi - psid/2, Controller/16(psid)
  Demux1/1 -> Controller/7(phi)

== system Quadcopter/single integrator/SquaDrone/Quadcopter3 ==
  xd : Inport
  yd : Inport  Port=2
  zd : Inport  Port=3
  psid : Inport  Port=4
  Controller : Subsystem
  Demux : Demux  Outputs=6
  Demux1 : Demux  Outputs=6
  Dynamic_System : Subsystem
  Mux : Mux  Inputs=6
  Mux1 : Mux  Inputs=6
  psi - psid : Scope  NumInputPorts=2
  x - xd : Scope  NumInputPorts=2
  y - yd : Scope  NumInputPorts=2
  z - zd : Scope  NumInputPorts=2
  x : Outport
  y : Outport  Port=2
  z : Outport  Port=3
  psi : Outport  Port=4
  wires:
  Dynamic_System/11(psi) -> psi/1, Mux1/5
  Controller/4(tau_psi) -> Dynamic_System/4(tau_psi)
  Dynamic_System/3(y) -> y/1, Mux/3
  Dynamic_System/1(x) -> x/1, Mux/1
  Controller/2(tau_phi) -> Dynamic_System/2(tau_phi)
  Dynamic_System/5(z) -> z/1, Mux/5
  Controller/3(tau_theta) -> Dynamic_System/3(tau_theta)
  Controller/1(Ft) -> Dynamic_System/1(Ft)
  Dynamic_System/2(dx) -> Mux/2
  Dynamic_System/4(dy) -> Mux/4
  Dynamic_System/6(dz) -> Mux/6
  Dynamic_System/7(phi) -> Mux1/1
  Dynamic_System/8(dphi) -> Mux1/2
  Dynamic_System/9(theta) -> Mux1/3
  Dynamic_System/10(dtheta) -> Mux1/4
  Dynamic_System/12(dpsi) -> Mux1/6
  Demux/1 -> x - xd/1, Controller/1(x)
  Demux/2 -> Controller/2(dx)
  Demux/3 -> y - yd/1, Controller/3(y)
  Demux/4 -> Controller/4(dy)
  Demux/5 -> Controller/5(z), z - zd/1
  Demux/6 -> Controller/6(dz)
  Mux/1 -> Demux/1
  Demux1/2 -> Controller/8(dphi)
  Demux1/3 -> Controller/9(theta)
  Demux1/4 -> Controller/10(dtheta)
  Demux1/5 -> psi - psid/1, Controller/11(psi)
  Demux1/6 -> Controller/12(dpsi)
  Mux1/1 -> Demux1/1
  xd/1 -> x - xd/2, Controller/13(xd)
  yd/1 -> y - yd/2, Controller/14(yd)
  zd/1 -> z - zd/2, Controller/15(zd)
  psid/1 -> psi - psid/2, Controller/16(psid)
  Demux1/1 -> Controller/7(phi)

== system Quadcopter/double integrator/SquaDrone/Drone1/Controller ==
  z : Inport
  dz : Inport  Port=2
  psi : Inport  Port=3
  dpsi : Inport  Port=4
  theta : Inport  Port=5
  dtheta : Inport  Port=6
  phi : Inport  Port=7
  dphi : Inport  Port=8
  zd : Inport  Port=9
  psid : Inport  Port=10
  thetad : Inport  Port=11
  dthetad : Inport  Port=12
  phid : Inport  Port=13
  dphid : Inport  Port=14
  Constant1 : Constant  Value=B_theta
  Constant14 : Constant  Value=B_z
  Constant20 : Constant  Value=B_psi
  Constant5 : Constant  Value=B_phi
  Gain{1,3,7..8} (4 alike) : Gain  Gain=2
  altitude : MATLAB Function  TreatAsAtomicUnit=on
  heading : MATLAB Function  TreatAsAtomicUnit=on
  lateral : MATLAB Function  TreatAsAtomicUnit=on
  longitudial : MATLAB Function  TreatAsAtomicUnit=on
  Ft : Outport
  tau_phi : Outport  Port=2
  tau_theta : Outport  Port=3
  tau_psi : Outport  Port=4
  wires:
  altitude/1(Ft) -> Ft/1
  longitudial/1(tau_phi) -> tau_phi/1
  lateral/1(tau_theta) -> tau_theta/1
  heading/1(tau_psi) -> tau_psi/1
  Gain7/1 -> altitude/7(M2)
  Constant14/1 -> Gain7/1, altitude/6(M1)
  Constant20/1 -> Gain8/1, heading/4(M1)
  Gain8/1 -> heading/5(M2)
  psid/1 -> heading/1(psid)
  psi/1 -> heading/2(psi)
  dpsi/1 -> heading/3(dpsi)
  theta/1 -> lateral/1(theta), altitude/4(theta)
  dtheta/1 -> lateral/2(dtheta)
  phi/1 -> longitudial/1(phi), altitude/3(phi)
  dphi/1 -> longitudial/2(dphi)
  zd/1 -> altitude/5(zd)
  z/1 -> altitude/1(z)
  dz/1 -> altitude/2(dz)
  Constant5/1 -> Gain3/1, longitudial/5(M1)
  Gain3/1 -> longitudial/6(M2)
  Constant1/1 -> Gain1/1, lateral/5(M1)
  Gain1/1 -> lateral/6(M2)
  thetad/1 -> lateral/3(thetad)
  dthetad/1 -> lateral/4(dthetad)
  phid/1 -> longitudial/3(phid)
  dphid/1 -> longitudial/4(dphid)
